simulink model "twolink_dynamic_model"  (R2017a)
settings: Solver=VariableStepAuto  StartTime=0.0  StopTime=10.0  RelTol=1e-3
settings Model: Creator=Zain  LastModifiedBy=Zain

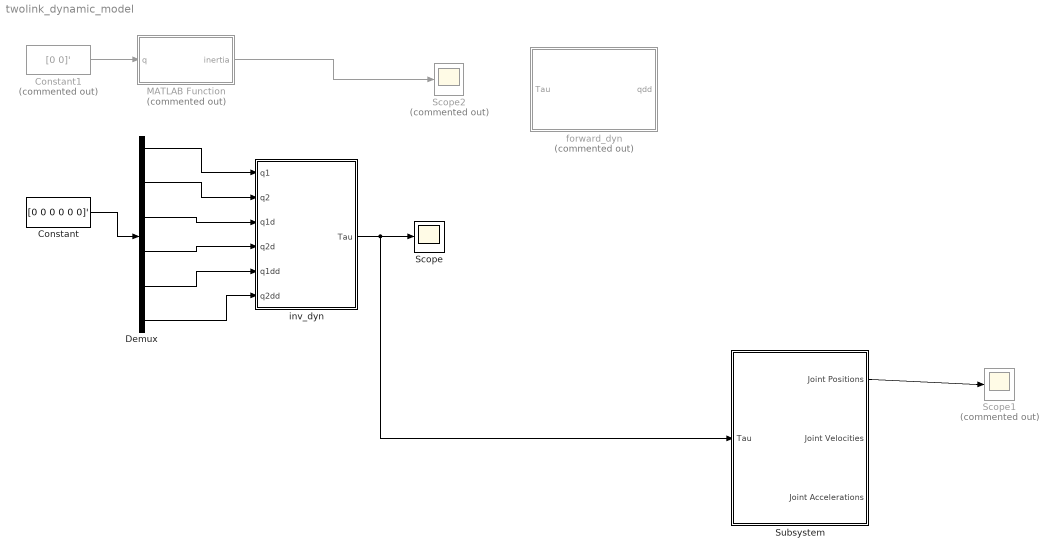
== system twolink_dynamic_model ==
  Constant : Constant  Value=[0 0 0 0 0 0]'
  Constant1 : Constant  Commented=on  Value=[0 0]'
  Demux : Demux  Outputs=6
  MATLAB Function : MATLAB Function  Commented=on  TreatAsAtomicUnit=on
  Scope : Scope
  Scope1 : Scope  Commented=on
  Scope2 : Scope  Commented=on
  Subsystem : Subsystem
  forward_dyn : MATLAB Function  Commented=on  TreatAsAtomicUnit=on
  inv_dyn : MATLAB Function  TreatAsAtomicUnit=on
  wires:
  inv_dyn/1(Tau) -> Subsystem/1(Tau), Scope/1
  Constant/1 -> Demux/1
  Demux/1 -> inv_dyn/1(q1)
  Demux/2 -> inv_dyn/2(q2)
  Demux/3 -> inv_dyn/3(q1d)
  Demux/4 -> inv_dyn/4(q2d)
  Demux/5 -> inv_dyn/5(q1dd)
  Demux/6 -> inv_dyn/6(q2dd)
  Subsystem/1(Joint Positions) -> Scope1/1
  Constant1/1 -> MATLAB Function/1(q)
  MATLAB Function/1(inertia) -> Scope2/1

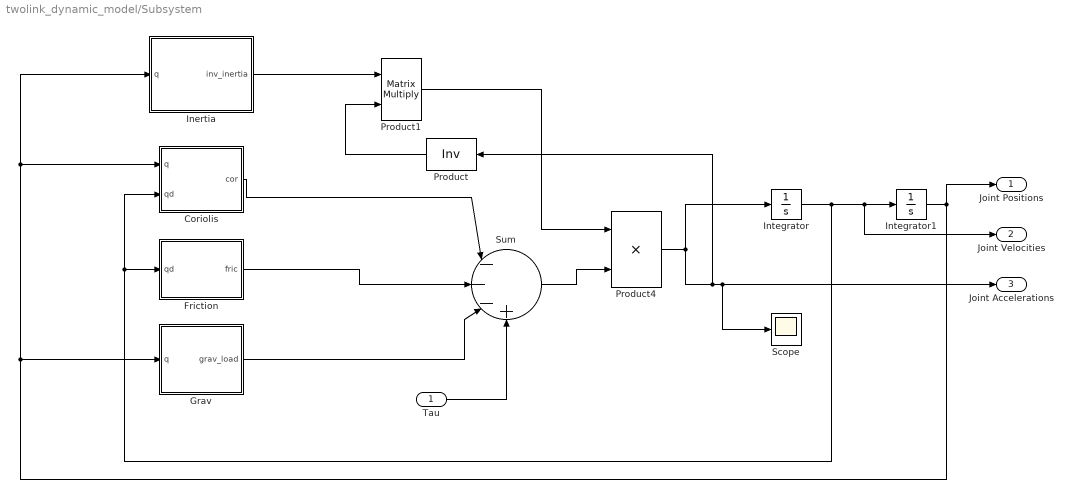
== system twolink_dynamic_model/Subsystem ==
  Tau : Inport
  Coriolis : MATLAB Function  TreatAsAtomicUnit=on
  Friction : MATLAB Function  TreatAsAtomicUnit=on
  Grav : MATLAB Function  TreatAsAtomicUnit=on
  Inertia : MATLAB Function  TreatAsAtomicUnit=on
  Integrator : Integrator
  Integrator1 : Integrator
  Product : Product  Inputs=/  Multiplication=Matrix(*)
  Product1 : Product  Multiplication=Matrix(*)
  Product4 : Product
  Scope : Scope
  Sum : Sum  Inputs=|---+
  Joint Positions : Outport
  Joint Velocities : Outport  Port=2
  Joint Accelerations : Outport  Port=3
  wires:
  Tau/1 -> Sum/4
  Coriolis/1(cor) -> Sum/1
  Friction/1(fric) -> Sum/2
  Grav/1(grav_load) -> Sum/3
  Integrator1/1 -> Joint Positions/1, Grav/1(q), Inertia/1(q), Coriolis/1(q)
  Integrator/1 -> Joint Velocities/1, Integrator1/1, Coriolis/2(qd), Friction/1(qd)
  Product4/1 -> Integrator/1, Product/1, Scope/1, Joint Accelerations/1
  Inertia/1(inv_inertia) -> Product1/1
  Product1/1 -> Product4/1
  Sum/1 -> Product4/2
  Product/1 -> Product1/2

== matlab function twolink_dynamic_model/forward_dyn ==
  data: Tau input; qdd output
function qdd = fcn(Tau)

m1= 1; m2= 1;
c1= 0.1; c2= 0.07;
a1= 0.2; a2= 0.15;
g= 9.81;
q1=0; q2=0;
q1d=0; q2d=0;
q1dd=0; q2dd=0;

Tau = [ m1*(a1 + c1)*(a1*q1dd + c1*q1dd + g*cos(q1)) + m2*(a2 + c2)*(a2*(q1dd + q2dd) + c2*(q1dd + q2dd) + cos(q2)*(a1*q1dd + g*cos(q1)) + sin(q2)*(a1*q1d^2 - g*sin(q1))) - a1*m2*sin(q2)*(a2*(q1d + q2d)^2 + c2*(q1d + q2d)^2 - sin(q2)*(a1*q1dd + g*cos(q1)) + cos(q2)*(a1*q1d^2 - g*sin(q1))) + a1*m2*cos(q2)*(a2*(q1dd + q2dd) + c2*(q1dd + q2dd) + cos(q2)*(a1*q1dd + g*cos(q1)) + sin(q2)*(a1*q1d^2 - g*sin(q1))); 
        m2*(a2 + c2)*(a2*(q1dd + q2dd) + c2*(q1dd + q2dd) + cos(q2)*(a1*q1dd + g*cos(q1)) + sin(q2)*(a1*q1d^2 - g*sin(q1)))];

inertia = [ m1*(a1 + c1)^2 + m2*(a2 + c2)*(a1 + a2 + c2) + a1*m2*(a1 + a2 + c2), m2*(a2 + c2)*(a1 + a2 + c2);
            m2*(a2 + c2)*(a1 + a2 + c2),              m2*(a2 + c2)^2];

        
        
cor =[ -a1*m2*q2d*sin(q2)*(a2 + c2), -a1*m2*sin(q2)*(a2 + c2)*(q1d + q2d);
        a1*m2*q1d*sin(q2)*(a2 + c2),                                   0];
         
        
gg = g*[q1 q2];
q_acc = (inertia)\(Tau-cor-gg);
qdd = q_acc(:,1);

== matlab function twolink_dynamic_model/inv_dyn ==
  data: q1 input; Tau output; q2 input; q1d input; q2d input; q1dd input; q2dd input
function Tau = fcn(q1,q2,q1d,q2d,q1dd,q2dd)
m1= 1; m2= 1;
c1= 0.1; c2= 0.07;
a1= 0.2; a2= 0.15;
g= 9.81;
% q1=0; q2=0;
% q1d=0; q2d=0;
% q1dd=0; q2dd=0;

Tau = [ m1*(a1 + c1)*(a1*q1dd + c1*q1dd + g*cos(q1)) + m2*(a2 + c2)*(a2*(q1dd + q2dd) + c2*(q1dd + q2dd) + cos(q2)*(a1*q1dd + g*cos(q1)) + sin(q2)*(a1*q1d^2 - g*sin(q1))) - a1*m2*sin(q2)*(a2*(q1d + q2d)^2 + c2*(q1d + q2d)^2 - sin(q2)*(a1*q1dd + g*cos(q1)) + cos(q2)*(a1*q1d^2 - g*sin(q1))) + a1*m2*cos(q2)*(a2*(q1dd + q2dd) + c2*(q1dd + q2dd) + cos(q2)*(a1*q1dd + g*cos(q1)) + sin(q2)*(a1*q1d^2 - g*sin(q1))), m2*(a2 + c2)*(a2*(q1dd + q2dd) + c2*(q1dd + q2dd) + cos(q2)*(a1*q1dd + g*cos(q1)) + sin(q2)*(a1*q1d^2 - g*sin(q1)))];

% tau1= Tau(1,1)
% tau2= Tau(1,2)

== matlab function twolink_dynamic_model/MATLAB Function ==
  data: q input; inertia output
function inertia = inert(q)
m1= 1; m2= 1;
c1= 0.1; c2= 0.07;
a1= 0.2; a2= 0.15;
inertia = [ m1*(a1 + c1)^2 + m2*(a2 + c2)*(a2 + c2 + a1*cos(q(2))) + a1^2*m2*sin(q(2))^2 + a1*m2*cos(q(2))*(a2 + c2 + a1*cos(q(2))), m2*(a2 + c2)*(a2 + c2 + a1*cos(q(2)));
                                                                        m2*(a2 + c2)^2 + a1*m2*cos(q(2))*(a2 + c2),                      m2*(a2 + c2)^2];

== matlab function twolink_dynamic_model/Subsystem/Coriolis ==
  data: q input; cor output; qd input
function cor = fcn(q,qd)
m1= 1; m2= 1;
c1= 0.1; c2= 0.07;
a1= 0.2; a2= 0.15;
cor = [ -a1*m2*qd(2)*sin(q(2))*(a2 + c2), -a1*m2*sin(q(2))*(a2 + c2)*(qd(1) + qd(2));
       a1*m2*qd(1)*sin(q(2))*(a2 + c2),                                    0];

== matlab function twolink_dynamic_model/Subsystem/Grav ==
  data: q input; grav_load output
function grav_load = grav(q)
m1= 1; m2= 1;
c1= 0.1; c2= 0.07;
a1= 0.2; a2= 0.15;
g= 9.81;

grav_load = [g*(a1*m1*cos(q(1)) + a1*m2*cos(q(1)) + c1*m1*cos(q(1)) + a2*m2*cos(q(1) + q(2)) + c2*m2*cos(q(1) + q(2))), g*m2*cos(q(1) + q(2))*(a2 + c2)];

== matlab function twolink_dynamic_model/Subsystem/Inertia ==
  data: q input; inv_inertia output
function inv_inertia = inv_iner(q)
m1= 1; m2= 1;
c1= 0.1; c2= 0.07;
a1= 0.2; a2= 0.15;

inv_inertia = [ m1*(a1 + c1)^2 + m2*(a2 + c2)*(a2 + c2 + a1*cos(q(2))) + a1^2*m2*sin(q(2))^2 + a1*m2*cos(q(2))*(a2 + c2 + a1*cos(q(2))), m2*(a2 + c2)*(a2 + c2 + a1*cos(q(2)));
                                                                       m2*(a2 + c2)^2 + a1*m2*cos(q(2))*(a2 + c2),                      m2*(a2 + c2)^2];
                                                                   
% inv_inertia = inv(inertia);
% inv_inertia1 = inv_inertia(:,1);

== matlab function twolink_dynamic_model/Subsystem/Friction ==
  data: qd input; fric output
function fric = friction_para(qd)
fric =[ -(37*qd(1))/25000, -(37*qd(2))/25000];
